simulink model "data_gen"  (R2018a)
settings: Solver=VariableStepAuto  StartTime=0.0  StopTime=SIMULATION_DURATION  FixedStep=0.0001  RelTol=1e-3
values from neighbouring files (symbols this model uses):
  DATA_SAMPLING_FREQUENCY = 500    [gymmed_test1.mat]    (also in simulation_setup.m; ws_1000_A0B0C0.mat)
settings Model: Creator=aaronrusso  LastModifiedBy=aaronrusso

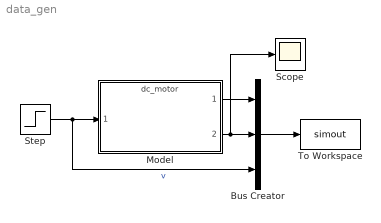
== system data_gen ==
  Bus Creator : BusCreator  Inputs=3
  Model : ModelReference  ModelNameDialog=dc_motor.slx  SimulationMode=Normal  ModelReferenceVersion=1.9
  Scope : Scope
  Step : Step  Time=0  After=5  SampleTime=0
  To Workspace : ToWorkspace  VariableName=simout  SaveFormat=Timeseries  SampleTime=1/DATA_SAMPLING_FREQUENCY
  wires:
  Step/1 -> Model/1, Bus Creator/3  "v"
  Model/1 -> Bus Creator/1
  Bus Creator/1 -> To Workspace/1
  Model/2 -> Scope/1, Bus Creator/2
